simulink model "untitledprotobackup"  (R2021b)
settings: Solver=ode15s  StartTime=0.0  StopTime=10  RelTol=1e-3
undefined symbols (not defined in the file): A, Ap, B1, B2x, Bp1, Bp2, C11, C12, C12a, C2, Cex, Cp2, Dp21, K1, K1a, K2, Lb, lmiganma, lmiganma3, nonlw, P, pAp1, pBp1, pCp1, strokedif
libraries: simulink x1
settings Model: Creator=ravi787  LastModifiedBy=ravi787
settings SolverCC: SolverResetMethod=Robust
settings DataIOCC: ExternalInput=[t, u,Adp,Bdp,Cdp,Ddp]  SaveState=on  ReturnWorkspaceOutputs=off
settings RTWCC: GenerateReport=on  LaunchReport=on

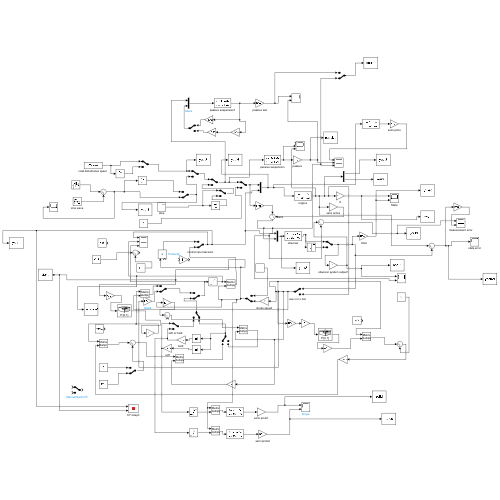
[thumbnail: Simulink's stored preview of the top-level diagram]
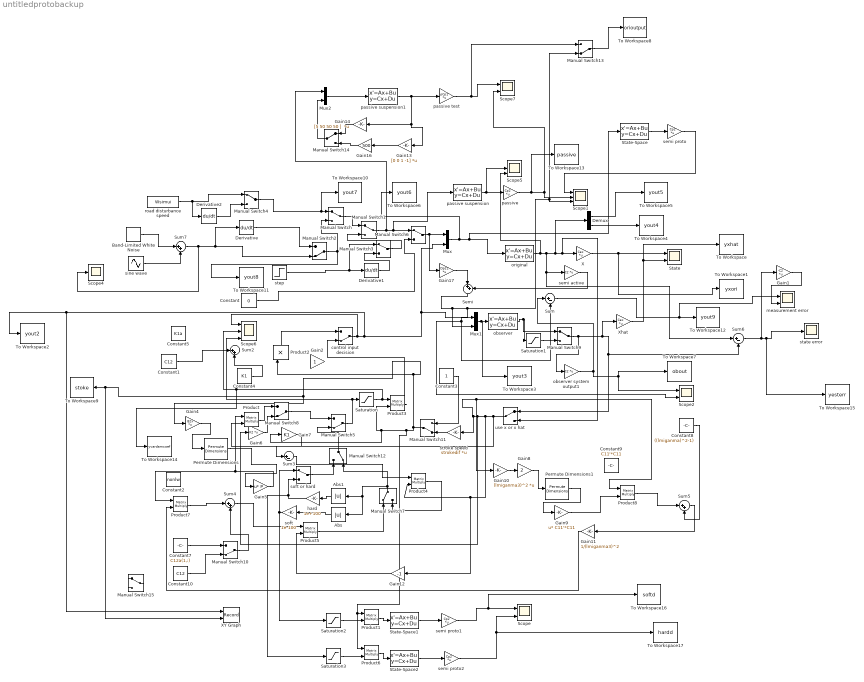
== system untitledprotobackup ==
  " soft" : Gain  Gain=1e-100  SampleTime=0.001
  Abs : Abs  SampleTime=0.001
  Abs1 : Abs  SampleTime=0.001
  Band-Limited White Noise : simulink/Sources/Band-Limited White Noise  Cov=[0.001]  Ts=0.001  seed=[23341]
  Constant : Constant  Value=0  SampleTime=0.001
  Constant1 : Constant  Value=C12  SampleTime=0.001
  Constant10 : Constant  Value=C12  SampleTime=0.001
  Constant2 : Constant  Value=nonlw  SampleTime=0.001
  Constant3 : Constant
  Constant4 : Constant  Value=K1  SampleTime=0.001
  Constant5 : Constant  Value=K1a
  Constant7 : Constant  Value=C12a(1,:)  SampleTime=0.001
  Constant8 : Constant  Value=((lmiganma)^2-1)  SampleTime=0.001
  Constant9 : Constant  Value=C11'*C11  SampleTime=0.001
  Demux : Demux  Outputs=2
  Derivative : Derivative
  Derivative1 : Derivative
  Derivative2 : Derivative
  Gain1 : Gain  Gain=-C2  Multiplication=Matrix(K*u)  SampleTime=0.001
  Gain10 : Gain  Gain=(lmiganma3)^2  Multiplication=Matrix(K*u)  SampleTime=0.001
  Gain11 : Gain  Gain=1/(lmiganma3)^2  SampleTime=0.001
  Gain12 : Gain  Gain=-1  SampleTime=0.001
  Gain13 : Gain  Gain=[0 0 1 -1]  Multiplication=Matrix(K*u)  SampleTime=0.001
  Gain14 : Gain  Gain=[5 50 50 50 ]  Multiplication=Matrix(K*u)  SampleTime=0.001
  Gain16 : Gain  Gain=500  SampleTime=0.001
  Gain17 : Gain  Gain=Dp21  Multiplication=Matrix(K*u)  SampleTime=0.001
  Gain2 : Gain
  Gain4 : Gain  Gain=B2x  Multiplication=Matrix(K*u)  SampleTime=0.001
  Gain5 : Gain  Gain=P  Multiplication=Matrix(u*K)  SampleTime=0.001
  Gain6 : Gain  Gain=K2  Multiplication=Matrix(K*u)  SampleTime=0.001
  Gain7 : Gain  Gain=K1  SampleTime=0.001
  Gain8 : Gain  Gain=2  SampleTime=0.001
  Gain9 : Gain  Gain=C11'*C11  Multiplication=Matrix(u*K)  SampleTime=0.001
  Manual Switch{,1,3..4,6..7,9,14} (8 alike) : ManualSwitch  SampleTime=0.001
  Manual Switch{2,5,8,10..13} (7 alike) : ManualSwitch  CurrentSetting=0  SampleTime=0.001
  Manual Switch15 : ManualSwitch
  Mux : Mux  Inputs=2
  Mux1 : Mux  Inputs=2
  Mux2 : Mux  Inputs=2
  Permute Dimensions : PermuteDimensions
  Permute Dimensions1 : PermuteDimensions
  Product{,1,3..8} (8 alike) : Product  Multiplication=Matrix(*)  SampleTime=0.001
  Product2 : Product  SampleTime=0.001
  Saturation : Saturate  UpperLimit=8000  LowerLimit=0  SampleTime=0.001
  Saturation1 : Saturate  UpperLimit=1000  LowerLimit=-1000  SampleTime=0.001
  Saturation2 : Saturate  UpperLimit=8000  LowerLimit=0  SampleTime=0.001
  Saturation3 : Saturate  UpperLimit=8000  LowerLimit=0  SampleTime=0.001
  Scope : Scope  NumInputPorts=2
  Scope1 : Scope  NumInputPorts=3
  Scope2 : Scope  NumInputPorts=2
  Scope4 : Scope
  Scope5 : Scope  NumInputPorts=3
  Scope6 : Scope  NumInputPorts=3
  Scope7 : Scope  NumInputPorts=2
  Semi : Sum  Inputs=|++  SampleTime=0.001
  State : Scope  NumInputPorts=2
  State-Space : StateSpace  A=Ap  B=[Bp1 Bp2]  C=eye(4)  D=zeros(4,2)  InitialCondition=0
  State-Space1 : StateSpace  A=Ap  B=[Bp1 Bp2]  C=eye(4)  D=zeros(4,2)  InitialCondition=0
  State-Space2 : StateSpace  A=Ap  B=[Bp1 Bp2]  C=eye(4)  D=zeros(4,2)  InitialCondition=0
  Sum : Sum  Inputs=|+-  SampleTime=0.001
  Sum{2,4..5,7} (4 alike) : Sum  Inputs=|++  SampleTime=0.001
  Sum3 : Sum  Inputs=|+-  SampleTime=0.001
  Sum6 : Sum  Inputs=|+-  SampleTime=0.001
  To Workspace : ToWorkspace  VariableName=yxhat  SampleTime=-1
      settings: Save2DSignal=2-D array (concatenate along first dimension)
  To Workspace1 : ToWorkspace  VariableName=yxori  SampleTime=-1
      settings: Save2DSignal=2-D array (concatenate along first dimension)
  To Workspace10 : ToWorkspace  VariableName=yout7  SampleTime=-1
      settings: Save2DSignal=2-D array (concatenate along first dimension)
  To Workspace11 : ToWorkspace  VariableName=yout8  SampleTime=-1
      settings: Save2DSignal=2-D array (concatenate along first dimension)
  To Workspace12 : ToWorkspace  VariableName=yout9  SampleTime=-1
      settings: Save2DSignal=2-D array (concatenate along first dimension)
  To Workspace13 : ToWorkspace  VariableName=passive  SampleTime=-1
      settings: Save2DSignal=2-D array (concatenate along first dimension)
  To Workspace14 : ToWorkspace  VariableName=yvardamcoef  SampleTime=-1
      settings: Save2DSignal=2-D array (concatenate along first dimension)
  To Workspace15 : ToWorkspace  VariableName=yesterr  SampleTime=0.001
  To Workspace16 : ToWorkspace  VariableName=softd  SampleTime=-1
      settings: Save2DSignal=2-D array (concatenate along first dimension)
  To Workspace17 : ToWorkspace  VariableName=hardd  SampleTime=-1
      settings: Save2DSignal=2-D array (concatenate along first dimension)
  To Workspace2 : ToWorkspace  VariableName=yout2  SampleTime=-1
      settings: Save2DSignal=2-D array (concatenate along first dimension)
  To Workspace3 : ToWorkspace  VariableName=yout3  SampleTime=-1
      settings: Save2DSignal=2-D array (concatenate along first dimension)
  To Workspace4 : ToWorkspace  VariableName=yout4  SampleTime=0.001
      settings: Save2DSignal=2-D array (concatenate along first dimension)
  To Workspace5 : ToWorkspace  VariableName=yout5  SampleTime=0.001
      settings: Save2DSignal=2-D array (concatenate along first dimension)
  To Workspace6 : ToWorkspace  VariableName=yout6  SampleTime=-1
      settings: Save2DSignal=2-D array (concatenate along first dimension)
  To Workspace7 : ToWorkspace  VariableName=obout  SampleTime=-1
      settings: Save2DSignal=2-D array (concatenate along first dimension)
  To Workspace8 : ToWorkspace  VariableName=orioutput  SampleTime=-1
      settings: Save2DSignal=2-D array (concatenate along first dimension)
  To Workspace9 : ToWorkspace  VariableName=stoke  SampleTime=-1
      settings: Save2DSignal=2-D array (concatenate along first dimension)
  X : Gain  Gain=Cex  Multiplication=Matrix(K*u)  SampleTime=0.001
  XY Graph : Record  FileSettingsInternal="{\"entries\":[{\"content\":{\"excelSettings\":{\"content\":{},\"type\":\"Streamout.ExcelSettings\"}},\"type\":\"Streamout.FileSettingStorage\",\"uuid\":\"e4f720ca-94c7-4a04-92da-525bd8d92d5f\"}],\"packageUris\":[\"http://schema.mathworks.com/mf0/streamout_blocks/R2020a\"],\"version\":\"1.0\"}"  Layout=[1 1]  SignalsInternal="{\"entries\":[{\"content\":{\"signals\":[{\"content\":{\"blockPath\":[\"untitledproto/XY Graph\"],\"channel\":[],\"dimensions\":[1],\"domain\":\"untitledproto/XY Graph\",\"lineColor\":\"#a2142f\",\"plots\":[1],\"port\":1,\"sid\":[\"\"],\"signalID\":122041,\"signalName\":\"control input decision\"},\"type\":\"RecordBlkView.Signal\",\"uuid\":\"db21bfa7-54c3-44fb-887d-2642e64da830\"},{\"content\":{\"blockPath\":[\"untitledproto/XY Graph\"],\"channel\":[],\"dimensions\":[1,1],\"domain\":\"untitledproto/XY Graph\",\"lineColor\":\"#139fff\",\"plots\":[1],\"port\":2,\"sid\":[\"\"],\"signalID\":122045,\"signalName\":\"Manual Switch11\"},\"type\":\"RecordBlkView.Signal\",\"uuid\":\"0a9d7882-ca07-4e7c-88a6-25abc54f678a\"}]},\"type\":\"RecordBlkView.InputSignals\",\"uuid\":\"6eaef8c5-dc51-4dfc-a136-ce674e642636\"}],\"packageUris\":[\"http://schema.mathworks.com/mf0/streamout_blocks/R2020a\"],\"version\":\"1.0\"}"  VisualizationBindings="{\"xyplotplugin\":{\"info\":[{\"series\":[{\"bindingParametersList\":[{\"parameter\":\"X-Axis\",\"signalID\":122045,\"signalName\":\"Manual Switch11\"},{\"parameter\":\"Y-Axis\",\"signalID\":122041,\"signalName\":\"control input decision\"}],\"seriesID\":47227}],\"subplotID\":1}]}}"  CompatibilityTag=XY
  Xhat : Gain  Gain=Cex  Multiplication=Matrix(K*u)  SampleTime=0.001
  control input decision : ManualSwitch  CurrentSetting=0  SampleTime=0.001
  "hard " : Gain  Gain=1e+100  SampleTime=0.001
  measurement error : Scope  NumInputPorts=2
  observer : StateSpace  A=(A+(Lb/10000)*C2)  B="[ B2x  -Lb/10000]"  C=eye(12)  D=zeros(12,4)  InitialCondition=0  ContinuousStateAttributes='observer'
  observer system output1 : Gain  Gain=C2  Multiplication=Matrix(K*u)  SampleTime=0.001
  original : StateSpace  A=A  B=[B1 B2x]  C=eye(12)  D=zeros(12,2)  InitialCondition=0  ParameterTunability=Unconstrained  ContinuousStateAttributes='original'
  passive : Gain  Gain=Cp2  Multiplication=Matrix(K*u)  SampleTime=0.001
  passive suspension : StateSpace  A=Ap  B=Bp1  C=eye(4)  D=zeros(4,1)  InitialCondition=0
  passive suspension1 : StateSpace  A=pAp1  B=[pBp1 Bp2]  C=eye(4)  D=zeros(4,2)  InitialCondition=0
  passive test : Gain  Gain=pCp1  Multiplication=Matrix(K*u)  SampleTime=0.001
  road disturbance speed : FromWorkspace  VariableName=Wsimui  OutDataTypeStr=double  SampleTime=0.001
  semi active : Gain  Gain=C2  Multiplication=Matrix(K*u)  SampleTime=0.001
  semi proto : Gain  Gain=Cp2  Multiplication=Matrix(K*u)  SampleTime=0.001
  semi proto1 : Gain  Gain=Cp2  Multiplication=Matrix(K*u)  SampleTime=0.001
  semi proto2 : Gain  Gain=Cp2  Multiplication=Matrix(K*u)  SampleTime=0.001
  sine wave : Sin  Frequency=5  SampleTime=0.001
  soft or hard : ManualSwitch  SampleTime=0.001
  state error : Scope
  step : Step  Time=0  SampleTime=0.001
  stroke speed : Gain  Gain=strokedif  Multiplication=Matrix(K*u)  SampleTime=0.001
  use x or x hat : ManualSwitch  SampleTime=0.001
  wires:
  observer/1 -> Manual Switch9/1, Saturation1/1
  Mux1/1 -> To Workspace3/1, observer/1
  original/1 -> Scope5/3, Sum6/1, semi active/1, use x or x hat/2, X/1, Demux/1
  Demux/2 -> To Workspace4/1
  Demux/1 -> To Workspace5/1
  Mux/1 -> To Workspace6/1, State-Space/1, original/1
  observer system output1/1 -> Sum/1, To Workspace7/1, Scope2/1
  Manual Switch/1 -> Manual Switch1/1
  Derivative/1 -> Manual Switch2/1
  Manual Switch2/1 -> Manual Switch/2, To Workspace11/1
  Manual Switch4/1 -> To Workspace10/1, Manual Switch/1
  step/1 -> Manual Switch3/1, Derivative1/1
  Derivative1/1 -> Manual Switch3/2
  Manual Switch3/1 -> Manual Switch1/2
  X/1 -> State/1, To Workspace1/1
  Xhat/1 -> State/2, To Workspace/1
  Sum/1 -> measurement error/1, To Workspace12/1
  road disturbance speed/1 -> Derivative2/1, Manual Switch4/1
  Derivative2/1 -> Manual Switch4/2
  semi active/1 -> Semi/2
  Semi/1 -> Mux1/2, Sum/2, Scope2/2, Manual Switch13/2, Scope1/3
  Manual Switch6/1 -> Mux/1, Gain17/1
  Constant/1 -> Manual Switch6/2
  Constant1/1 -> Sum2/1
  passive suspension/1 -> Scope5/2, passive/1
  passive/1 -> To Workspace13/1, Scope7/2, Scope1/2
  Permute Dimensions/1 -> Gain5/1
  Manual Switch11/1 -> Product6/1, Product1/1, Gain7/1, Product3/2, XY Graph/2, To Workspace9/1, Gain4/1, Product2/1
  Gain4/1 -> Permute Dimensions/1
  Constant4/1 -> Sum2/2
  Product2/1 -> control input decision/1
  control input decision/1 -> Scope6/1, To Workspace2/1, XY Graph/1, Mux/2, Mux1/1
  Gain7/1 -> Sum3/1
  Sum3/1 -> Product4/1
  Product5/1 -> Manual Switch7/1
  Product4/1 -> Manual Switch7/2
  Sum4/1 -> Product5/1
  Gain10/1 -> Gain8/1
  Constant8/1 -> Sum5/2
  Sum5/1 -> Gain11/1
  Product7/1 -> Sum4/1
  Gain5/1 -> Product7/1, Product/1
  Gain11/1 -> Product7/2
  use x or x hat/1 -> Product/2, stroke speed/1, Product8/1, Gain10/1, Gain6/1, Gain12/1, Product4/2
  Product8/1 -> Sum5/1
  Gain8/1 -> Permute Dimensions1/1
  Permute Dimensions1/1 -> Gain9/1
  Gain9/1 -> Product8/2
  Gain6/1 -> Manual Switch8/2
  Product/1 -> Manual Switch8/1
  Manual Switch8/1 -> Manual Switch5/1
  Saturation/1 -> Scope6/2, To Workspace14/1, Product3/1
  Manual Switch5/1 -> Scope6/3, Saturation/1
  Sum6/1 -> Gain1/1, To Workspace15/1, state error/1
  Saturation1/1 -> Manual Switch9/2
  Manual Switch9/1 -> observer system output1/1, Xhat/1, Sum6/2, use x or x hat/1
  Gain12/1 -> Product5/2
  Constant7/1 -> Manual Switch10/1
  Constant10/1 -> Manual Switch10/2
  Manual Switch10/1 -> Sum4/2
  stroke speed/1 -> Manual Switch11/2
  Constant3/1 -> Manual Switch11/1
  Gain1/1 -> measurement error/2
  Manual Switch12/1 -> Manual Switch5/2
  Abs/1 -> " soft"/1
  Manual Switch7/1 -> Manual Switch12/2, Abs1/1, Abs/1
  soft or hard/1 -> Manual Switch12/1
  " soft"/1 -> soft or hard/1, Saturation2/1
  Abs1/1 -> "hard "/1
  "hard "/1 -> Saturation3/1, soft or hard/2
  Band-Limited White Noise/1 -> Sum7/1
  sine wave/1 -> Sum7/2
  Sum7/1 -> Scope4/1, Derivative/1, Manual Switch2/2
  Product3/1 -> control input decision/2
  Manual Switch1/1 -> Mux2/1, Manual Switch6/1, passive suspension/1
  passive suspension1/1 -> Gain13/1, Gain14/1, passive test/1
  Mux2/1 -> passive suspension1/1
  passive test/1 -> Manual Switch13/1, Scope7/1
  Manual Switch13/1 -> To Workspace8/1
  Gain14/1 -> Manual Switch14/1
  Manual Switch14/1 -> Mux2/2
  Gain16/1 -> Manual Switch14/2
  Gain13/1 -> Gain16/1
  Gain17/1 -> Semi/1
  State-Space/1 -> semi proto/1
  semi proto/1 -> Scope1/1
  State-Space1/1 -> semi proto1/1
  State-Space2/1 -> semi proto2/1
  Saturation3/1 -> Product6/2
  Saturation2/1 -> Product1/2
  Product1/1 -> State-Space1/1
  Product6/1 -> State-Space2/1
  semi proto1/1 -> To Workspace16/1, Scope/1
  semi proto2/1 -> To Workspace17/1, Scope/2
